simulink model "Test_MIMO"  (R2020a)
settings: Solver=FixedStepAuto  StartTime=0.0  StopTime=10.0  FixedStep=0.1  MaxStep=0.1  RelTol=1e-3
undefined symbols (not defined in the file or in its folder): DiscIntNeverNeededParam
Description:
  | A simple model
settings Model: DataDictionary=TestConfig.sldd  Creator=raarenst  LastModifiedBy=toma
settings OptimizationCC: DefaultParameterBehavior=Inlined  EnhancedBackFolding=on  PassReuseOutputArgsAs=Individual arguments  ZeroExternalMemoryAtStartup=off  ZeroInternalMemoryAtStartup=off  OptimizeBlockOrder=speed  DifferentSizesBufferReuse=on  OptimizationCustomize=off  EfficientTunableParamExpr=on
settings DebuggingCC: UnderspecifiedInitializationDetection=Classic  MergeDetectMultiDrivingBlocksExec=none  ParameterTunabilityLossMsg=error  ModelReferenceSymbolNameMessage=none
settings ModelReferenceCC: PropagateSignalLabelsOutOfModel=off
settings SFSimCC: MATLABDynamicMemAlloc=off
settings RTWCC: Description=CIGRE export target  SystemTargetFile=cigre.tlc  TemplateMakefile=cigre_tmf  Toolchain=CIGRE DLL - Microsoft Visual C++ 2019 (64bit) | nmake makefile (64-bit Windows)
settings CodeAppCC: ForceParamTrailComments=on  IgnoreCustomStorageClasses=off  OperatorAnnotations=on  SimulinkDataObjDesc=on  SFDataObjDesc=on  InsertBlockDesc=on
settings STFCustomTargetCC: TargetLangStandard=C99 (ISO)  MultiwordLength=256  GenerateSampleERTMain=on  CompOptLevelCompliant=on  CombineOutputUpdateFcns=on  ERTCustomFileBanners=on  MultiInstanceERTCode=on  CodeInterfacePackaging=Reusable function  SupportContinuousTime=off  SupportNonInlinedSFcns=off  RemoveResetFunc=on  MATLABClassNameForMDSCustomization=Simulink.SoftwareTarget.ERTCustomization  UseToolchainInfoCompliant=on  SystemTargetFile=cigre.tlc
settings ERTTargetCC: TargetLangStandard=C99 (ISO)  GenerateSampleERTMain=on  ParMdlRefBuildCompliant=off  ConcurrentExecutionCompliant=off  MultiInstanceERTCode=on  CodeInterfacePackaging=Reusable function  ModelStepFunctionPrototypeControlCompliant=off  CPPClassGenCompliant=off  InlinedParameterPlacement=NonHierarchical  RootIOFormat=Structure reference  ERTCustomFileTemplate=example_file_process.tlc

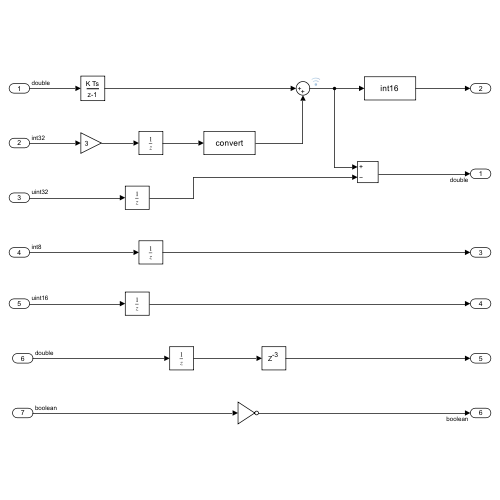
[thumbnail: Simulink's stored preview of the top-level diagram]
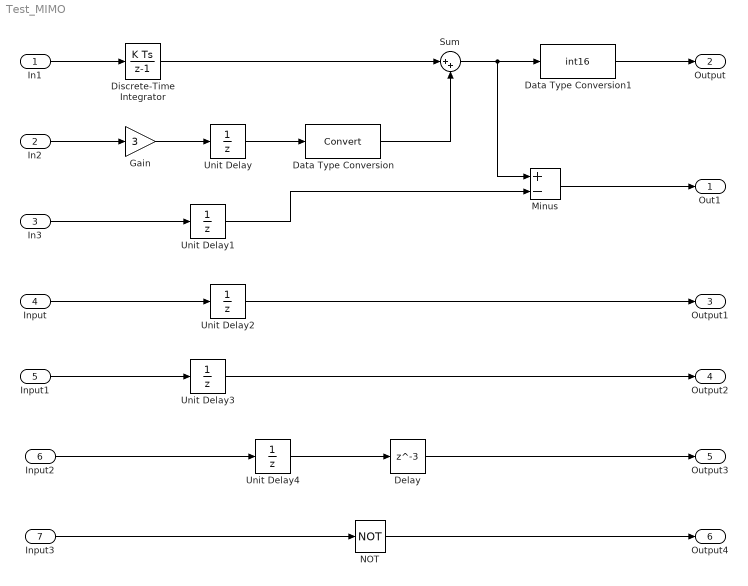
== system Test_MIMO ==
  In1 : Inport  OutDataTypeStr=double  SampleTime=0.1
  In2 : Inport  Port=2  OutDataTypeStr=int32  SampleTime=0.1
  In3 : Inport  Port=3  OutDataTypeStr=uint32
  Input : Inport  Port=4  OutDataTypeStr=int8
  Input1 : Inport  Port=5  OutDataTypeStr=uint16
  Input2 : Inport  Port=6  OutDataTypeStr=double
  Input3 : Inport  Port=7  OutDataTypeStr=boolean
  Data Type Conversion : DataTypeConversion
  Data Type Conversion1 : DataTypeConversion  OutDataTypeStr=int16
  Delay : Delay  DelayLength=3
  Discrete-Time Integrator : DiscreteIntegrator  SampleTime=-1  ICPrevOutput=DiscIntNeverNeededParam  ICPrevScaledInput=DiscIntNeverNeededParam
  Gain : Gain  Gain=3  OutDataTypeStr=int32
  Minus : Sum  Inputs=+-
  NOT : Logic  Operator=NOT  IconShape=distinctive  AllPortsSameDT=off  OutDataTypeStr=boolean
  Sum : Sum  Inputs=|++
  Unit Delay : UnitDelay  SampleTime=-1  HasFrameUpgradeWarning=on
  Unit Delay1 : UnitDelay  SampleTime=-1  HasFrameUpgradeWarning=on
  Unit Delay2 : UnitDelay  SampleTime=-1  HasFrameUpgradeWarning=on
  Unit Delay3 : UnitDelay  InitialCondition=1  SampleTime=-1  HasFrameUpgradeWarning=on
  Unit Delay4 : UnitDelay  InitialCondition=2  SampleTime=-1  HasFrameUpgradeWarning=on
  Out1 : Outport  OutDataTypeStr=double
  Output : Outport  Port=2
  Output1 : Outport  Port=3
  Output2 : Outport  Port=4
  Output3 : Outport  Port=5
  Output4 : Outport  Port=6  OutDataTypeStr=boolean
  wires:
  In2/1 -> Gain/1
  Gain/1 -> Unit Delay/1
  Unit Delay/1 -> Data Type Conversion/1
  In1/1 -> Discrete-Time Integrator/1
  Data Type Conversion/1 -> Sum/2
  Discrete-Time Integrator/1 -> Sum/1
  Sum/1 -> Minus/1, Data Type Conversion1/1
  Minus/1 -> Out1/1
  In3/1 -> Unit Delay1/1
  Data Type Conversion1/1 -> Output/1
  Input/1 -> Unit Delay2/1
  Input1/1 -> Unit Delay3/1
  Input2/1 -> Unit Delay4/1
  Unit Delay1/1 -> Minus/2
  Unit Delay2/1 -> Output1/1
  Unit Delay3/1 -> Output2/1
  Unit Delay4/1 -> Delay/1
  Delay/1 -> Output3/1
  Input3/1 -> NOT/1
  NOT/1 -> Output4/1
